simulink library "haley_test_bench_lib"  (Simulink 9.2)
settings: Solver=VariableStepAuto  StartTime=0.0  StopTime=10.0  RelTol=1e-3
undefined symbols (not defined in the file or in its folder): p_max_bar, t_sample_s
libraries: etherlab_lib x4, powerlib_meascontrol x2, simulink x1, pePwmGenerator x1
settings Model: Creator=habich  LastModifiedBy=entwicklungs-pc

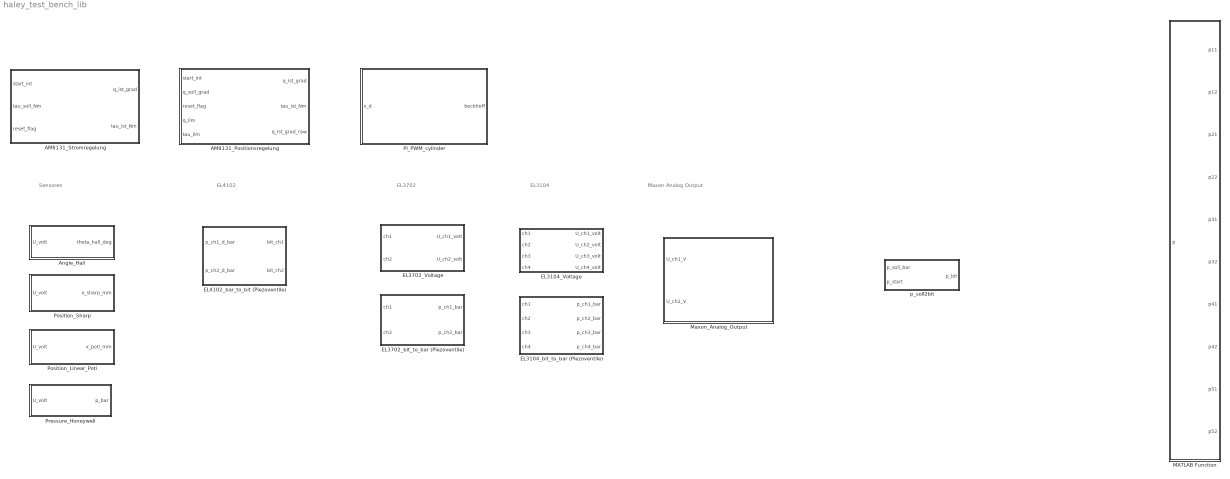
== system haley_test_bench_lib ==
  note: Sensoren
  note: EL4102
  note: EL3702
  note: Maxon Analog Output
  note: EL3104
  AM8131_Positionsregelung : Subsystem
  AM8131_Stromregelung : Subsystem
  Angle_Hall : MATLAB Function  TreatAsAtomicUnit=on
  EL3104_Voltage : Subsystem
  EL3104_bit_to_bar (Piezoventile) : Subsystem
  EL3702_Voltage : Subsystem
  EL3702_bit_to_bar (Piezoventile) : Subsystem
  EL4102_bar_to_bit (Piezoventile) : MATLAB Function  TreatAsAtomicUnit=on
  MATLAB Function : MATLAB Function  TreatAsAtomicUnit=on
  Maxon_Analog_Output : Subsystem
  PI_PWM_cylinder : Subsystem
  "Position_Linear_Poti " : MATLAB Function  TreatAsAtomicUnit=on
  Position_Sharp : MATLAB Function  TreatAsAtomicUnit=on
  Pressure_Honeywell : MATLAB Function  TreatAsAtomicUnit=on
  p_soll2bit : Subsystem

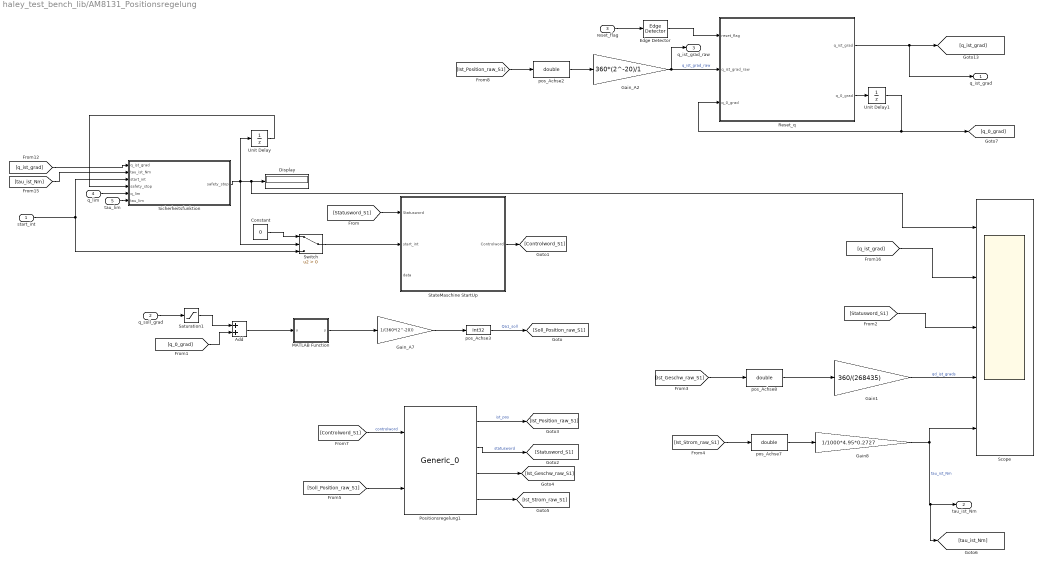
== system haley_test_bench_lib/AM8131_Positionsregelung ==
  start_int : Inport
  q_soll_grad : Inport  Port=2
  "reset_flag " : Inport  Port=3
  q_lim : Inport  Port=4
  tau_lim : Inport  Port=5
  Add : Sum
  Constant : Constant  Value=0
  Display : Display
  Edge Detector : powerlib_meascontrol/Logic/Edge Detector  model=Rising  ic=0  Ts=1e-3
      settings: SourceProductName=Simscape Electrical  SourceProductBaseCode=PS
  Gain1 : Gain  Gain=360/(268435)
  Gain8 : Gain  Gain=1/1000*4.95*0.2727
  Gain_A2 : Gain  Gain=360*(2^-20)/1
  Gain_A7 : Gain  Gain=1/(360*(2^-20))
  MATLAB Function : MATLAB Function  TreatAsAtomicUnit=on
  Positionsregelung1 : etherlab_lib/EtherCAT/Generic_0  master=0  index=6  rv=slave_el7211_pos  param=[]  tsample=0.001  debug=0
  Reset_q : MATLAB Function  TreatAsAtomicUnit=on
  Saturation1 : Saturate  UpperLimit=5  LowerLimit=-5
  Scope : Scope  NumInputPorts=5
  Sicherheitsfunktion : MATLAB Function  TreatAsAtomicUnit=on
  StateMaschine StartUp : Stateflow chart  TreatAsAtomicUnit=on
  Switch : Switch  Criteria=u2 > Threshold
  Unit Delay : UnitDelay  SampleTime=1e-3
  Unit Delay1 : UnitDelay  SampleTime=1e-3
  pos_Achse2 : DataTypeConversion  OutDataTypeStr=double
  pos_Achse3 : DataTypeConversion  OutDataTypeStr=int32
  pos_Achse7 : DataTypeConversion  OutDataTypeStr=double
  pos_Achse8 : DataTypeConversion  OutDataTypeStr=double
  "q_ist_grad " : Outport
  tau_ist_Nm : Outport  Port=2
  q_ist_grad_raw : Outport  Port=3
  wires:
  Positionsregelung1/1 -> [Ist_Position_raw_S1]  "ist_pos"
  [Statusword_S1] -> StateMaschine StartUp/1(Statusword)
  [Ist_Strom_raw_S1] -> pos_Achse7/1
  pos_Achse7/1 -> Gain8/1
  Positionsregelung1/2 -> [Statusword_S1]  "statusword"
  Gain8/1 -> [tau_ist_Nm], tau_ist_Nm/1, Scope/5  "tau_ist_Nm"
  StateMaschine StartUp/1(Controlword) -> [Controlword_S1]
  [Controlword_S1] -> Positionsregelung1/1  "controlword"
  [Statusword_S1] -> Scope/3
  Positionsregelung1/3 -> [Ist_Geschw_raw_S1]
  pos_Achse8/1 -> Gain1/1
  [Ist_Geschw_raw_S1] -> pos_Achse8/1
  Gain1/1 -> Scope/4  "qd_ist_grads"
  Positionsregelung1/4 -> [Ist_Strom_raw_S1]
  MATLAB Function/1(y) -> Gain_A7/1
  q_soll_grad/1 -> Saturation1/1
  Add/1 -> MATLAB Function/1(u)
  [Soll_Position_raw_S1] -> Positionsregelung1/2
  Gain_A7/1 -> pos_Achse3/1
  pos_Achse3/1 -> [Soll_Position_raw_S1]  "Qa1_soll"
  Reset_q/1(q_ist_grad) -> "q_ist_grad "/1, [q_ist_grad]
  [Ist_Position_raw_S1] -> pos_Achse2/1
  "reset_flag "/1 -> Edge Detector/1
  Edge Detector/1 -> Reset_q/1(reset_flag)
  Gain_A2/1 -> Reset_q/2(q_ist_grad_raw), q_ist_grad_raw/1  "q_ist_grad_raw"
  Reset_q/2(q_0_grad) -> Unit Delay1/1
  pos_Achse2/1 -> Gain_A2/1
  Unit Delay1/1 -> Reset_q/3("q_0_grad "), [q_0_grad]
  [q_ist_grad] -> Scope/2
  Unit Delay/1 -> Sicherheitsfunktion/4("safety_stop ")
  [q_ist_grad] -> Sicherheitsfunktion/1(q_ist_grad)
  Constant/1 -> Switch/1
  start_int/1 -> Switch/3, Sicherheitsfunktion/3(start_int)
  Sicherheitsfunktion/1(safety_stop) -> Scope/1, Display/1, Switch/2, Unit Delay/1
  [tau_ist_Nm] -> Sicherheitsfunktion/2(tau_ist_Nm)
  Switch/1 -> StateMaschine StartUp/2(start_int)
  [q_0_grad] -> Add/2
  Saturation1/1 -> Add/1
  q_lim/1 -> Sicherheitsfunktion/5(q_lim)
  tau_lim/1 -> Sicherheitsfunktion/6(tau_lim)

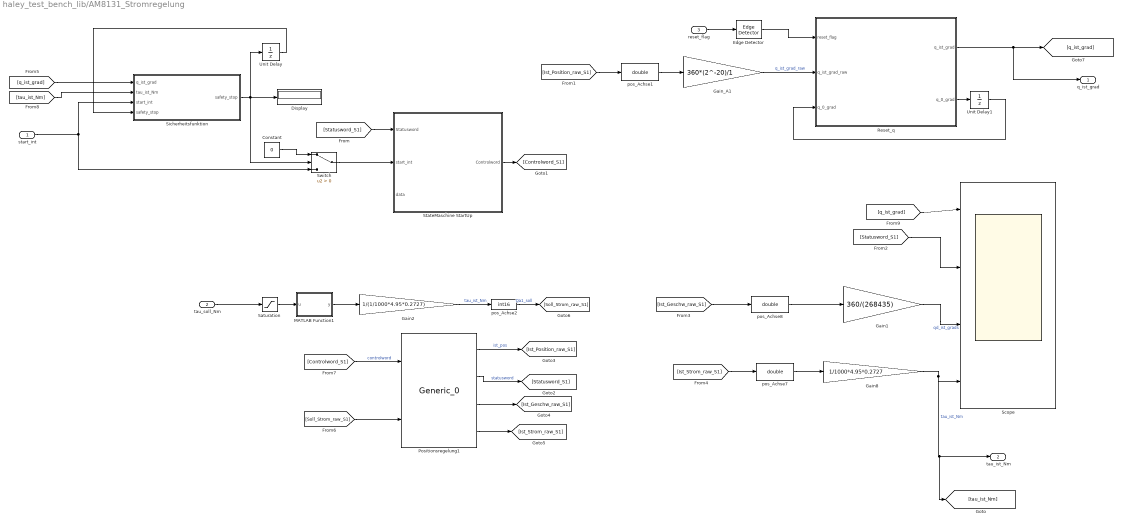
== system haley_test_bench_lib/AM8131_Stromregelung ==
  start_int : Inport
  tau_soll_Nm : Inport  Port=2
  "reset_flag " : Inport  Port=3
  Constant : Constant  Value=0
  Display : Display
  Edge Detector : powerlib_meascontrol/Logic/Edge Detector  model=Rising  ic=0  Ts=1e-3
      settings: SourceProductName=Simscape Electrical  SourceProductBaseCode=PS
  Gain1 : Gain  Gain=360/(268435)
  Gain2 : Gain  Gain=1/(1/1000*4.95*0.2727)
  Gain8 : Gain  Gain=1/1000*4.95*0.2727
  Gain_A1 : Gain  Gain=360*(2^-20)/1
  MATLAB Function1 : MATLAB Function  TreatAsAtomicUnit=on
  Positionsregelung1 : etherlab_lib/EtherCAT/Generic_0  master=0  index=6  rv=slave_el7211_strom  param=[]  tsample=0.001  debug=0
  Reset_q : MATLAB Function  TreatAsAtomicUnit=on
  Saturation : Saturate
  Scope : Scope  NumInputPorts=4
  Sicherheitsfunktion : MATLAB Function  TreatAsAtomicUnit=on
  StateMaschine StartUp : Stateflow chart  TreatAsAtomicUnit=on
  Switch : Switch  Criteria=u2 > Threshold
  Unit Delay : UnitDelay  SampleTime=1e-3
  Unit Delay1 : UnitDelay  SampleTime=1e-3
  pos_Achse1 : DataTypeConversion  OutDataTypeStr=double
  pos_Achse2 : DataTypeConversion  OutDataTypeStr=int16
  pos_Achse7 : DataTypeConversion  OutDataTypeStr=double
  pos_Achse8 : DataTypeConversion  OutDataTypeStr=double
  "q_ist_grad " : Outport
  "tau_ist_Nm " : Outport  Port=2
  wires:
  [Ist_Position_raw_S1] -> pos_Achse1/1
  Positionsregelung1/1 -> [Ist_Position_raw_S1]  "ist_pos"
  [Statusword_S1] -> StateMaschine StartUp/1(Statusword)
  [Ist_Strom_raw_S1] -> pos_Achse7/1
  pos_Achse7/1 -> Gain8/1
  MATLAB Function1/1(y) -> Gain2/1
  pos_Achse1/1 -> Gain_A1/1
  Positionsregelung1/2 -> [Statusword_S1]  "statusword"
  Gain8/1 -> [tau_ist_Nm], "tau_ist_Nm "/1, Scope/4  "tau_ist_Nm"
  StateMaschine StartUp/1(Controlword) -> [Controlword_S1]
  Saturation/1 -> MATLAB Function1/1(u)
  start_int/1 -> Switch/3, Sicherheitsfunktion/3(start_int)
  tau_soll_Nm/1 -> Saturation/1
  Gain2/1 -> pos_Achse2/1  "tau_ist_Nm"
  [Soll_Strom_raw_S1] -> Positionsregelung1/2
  [Controlword_S1] -> Positionsregelung1/1  "controlword"
  [Statusword_S1] -> Scope/2
  Positionsregelung1/3 -> [Ist_Geschw_raw_S1]
  pos_Achse8/1 -> Gain1/1
  [Ist_Geschw_raw_S1] -> pos_Achse8/1
  Gain1/1 -> Scope/3  "qd_ist_grads"
  Positionsregelung1/4 -> [Ist_Strom_raw_S1]
  pos_Achse2/1 -> [Soll_Strom_raw_S1]  "Qa1_soll"
  [q_ist_grad] -> Sicherheitsfunktion/1(q_ist_grad)
  [tau_ist_Nm] -> Sicherheitsfunktion/2(tau_ist_Nm)
  Sicherheitsfunktion/1(safety_stop) -> Display/1, Switch/2, Unit Delay/1
  Unit Delay/1 -> Sicherheitsfunktion/4("safety_stop ")
  Constant/1 -> Switch/1
  Switch/1 -> StateMaschine StartUp/2(start_int)
  Edge Detector/1 -> Reset_q/1(reset_flag)
  Gain_A1/1 -> Reset_q/2(q_ist_grad_raw)  "q_ist_grad_raw"
  Reset_q/2(q_0_grad) -> Unit Delay1/1
  Unit Delay1/1 -> Reset_q/3("q_0_grad ")
  Reset_q/1(q_ist_grad) -> "q_ist_grad "/1, [q_ist_grad]
  [q_ist_grad] -> Scope/1
  "reset_flag "/1 -> Edge Detector/1

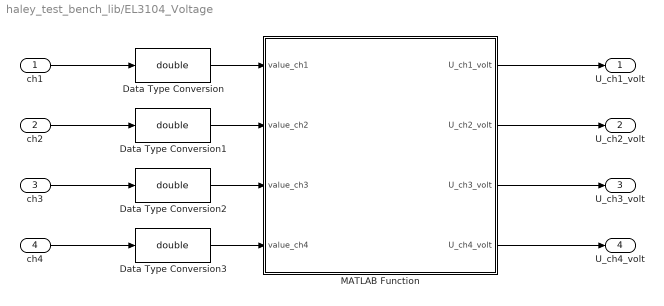
== system haley_test_bench_lib/EL3104_Voltage ==
  ch1 : Inport
  ch2 : Inport  Port=2
  ch3 : Inport  Port=3
  ch4 : Inport  Port=4
  Data Type Conversion{,1..3} (4 alike) : DataTypeConversion  OutDataTypeStr=double
  MATLAB Function : MATLAB Function  TreatAsAtomicUnit=on
  U_ch1_volt : Outport
  U_ch2_volt : Outport  Port=2
  U_ch3_volt : Outport  Port=3
  U_ch4_volt : Outport  Port=4
  wires:
  ch1/1 -> Data Type Conversion/1
  ch2/1 -> Data Type Conversion1/1
  Data Type Conversion1/1 -> MATLAB Function/2(value_ch2)
  MATLAB Function/2(U_ch2_volt) -> U_ch2_volt/1
  Data Type Conversion/1 -> MATLAB Function/1(value_ch1)
  MATLAB Function/1(U_ch1_volt) -> U_ch1_volt/1
  Data Type Conversion2/1 -> MATLAB Function/3(value_ch3)
  ch3/1 -> Data Type Conversion2/1
  Data Type Conversion3/1 -> MATLAB Function/4(value_ch4)
  ch4/1 -> Data Type Conversion3/1
  MATLAB Function/3(U_ch3_volt) -> U_ch3_volt/1
  MATLAB Function/4(U_ch4_volt) -> U_ch4_volt/1

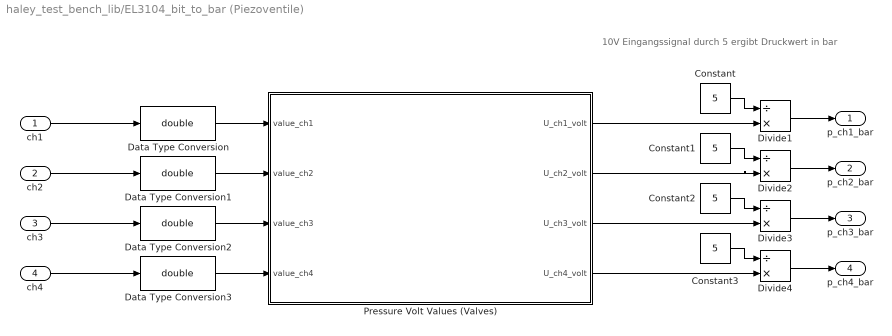
== system haley_test_bench_lib/EL3104_bit_to_bar (Piezoventile) ==
  note: 10V Eingangssignal durch 5 ergibt Druckwert in bar
  ch1 : Inport
  ch2 : Inport  Port=2
  ch3 : Inport  Port=3
  ch4 : Inport  Port=4
  Constant{,1..3} (4 alike) : Constant  Value=5
  Data Type Conversion{,1..3} (4 alike) : DataTypeConversion  OutDataTypeStr=double
  Divide{1..4} (4 alike) : Product  Inputs=/*
  Pressure Volt Values (Valves) : MATLAB Function  TreatAsAtomicUnit=on
  p_ch1_bar : Outport
  p_ch2_bar : Outport  Port=2
  p_ch3_bar : Outport  Port=3
  p_ch4_bar : Outport  Port=4
  wires:
  Pressure Volt Values (Valves)/1(U_ch1_volt) -> Divide1/2
  Constant/1 -> Divide1/1
  Data Type Conversion1/1 -> Pressure Volt Values (Valves)/2(value_ch2)
  Divide1/1 -> p_ch1_bar/1
  ch2/1 -> Data Type Conversion1/1
  ch1/1 -> Data Type Conversion/1
  Data Type Conversion/1 -> Pressure Volt Values (Valves)/1(value_ch1)
  Data Type Conversion2/1 -> Pressure Volt Values (Valves)/3(value_ch3)
  ch3/1 -> Data Type Conversion2/1
  Data Type Conversion3/1 -> Pressure Volt Values (Valves)/4(value_ch4)
  ch4/1 -> Data Type Conversion3/1
  Pressure Volt Values (Valves)/2(U_ch2_volt) -> Divide2/2
  Divide2/1 -> p_ch2_bar/1
  Constant1/1 -> Divide2/1
  Pressure Volt Values (Valves)/3(U_ch3_volt) -> Divide3/2
  Divide3/1 -> p_ch3_bar/1
  Constant2/1 -> Divide3/1
  Pressure Volt Values (Valves)/4(U_ch4_volt) -> Divide4/2
  Divide4/1 -> p_ch4_bar/1
  Constant3/1 -> Divide4/1

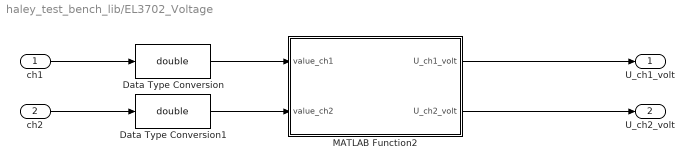
== system haley_test_bench_lib/EL3702_Voltage ==
  "ch1 " : Inport
  ch2 : Inport  Port=2
  Data Type Conversion : DataTypeConversion  OutDataTypeStr=double
  Data Type Conversion1 : DataTypeConversion  OutDataTypeStr=double
  MATLAB Function2 : MATLAB Function  TreatAsAtomicUnit=on
  U_ch1_volt : Outport
  U_ch2_volt : Outport  Port=2
  wires:
  MATLAB Function2/1(U_ch1_volt) -> U_ch1_volt/1
  Data Type Conversion1/1 -> MATLAB Function2/2(value_ch2)
  ch2/1 -> Data Type Conversion1/1
  "ch1 "/1 -> Data Type Conversion/1
  Data Type Conversion/1 -> MATLAB Function2/1(value_ch1)
  MATLAB Function2/2(U_ch2_volt) -> U_ch2_volt/1

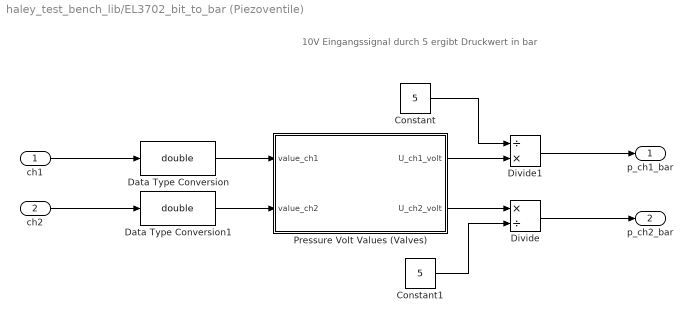
== system haley_test_bench_lib/EL3702_bit_to_bar (Piezoventile) ==
  note: 10V Eingangssignal durch 5 ergibt Druckwert in bar
  "ch1 " : Inport
  ch2 : Inport  Port=2
  Constant : Constant  Value=5
  Constant1 : Constant  Value=5
  Data Type Conversion : DataTypeConversion  OutDataTypeStr=double
  Data Type Conversion1 : DataTypeConversion  OutDataTypeStr=double
  Divide : Product  Inputs=*/
  Divide1 : Product  Inputs=/*
  Pressure Volt Values (Valves) : MATLAB Function  TreatAsAtomicUnit=on
  p_ch1_bar : Outport
  p_ch2_bar : Outport  Port=2
  wires:
  "ch1 "/1 -> Data Type Conversion/1
  Pressure Volt Values (Valves)/2(U_ch2_volt) -> Divide/1
  ch2/1 -> Data Type Conversion1/1
  Pressure Volt Values (Valves)/1(U_ch1_volt) -> Divide1/2
  Constant/1 -> Divide1/1
  Divide1/1 -> p_ch1_bar/1
  Divide/1 -> p_ch2_bar/1
  Constant1/1 -> Divide/2
  Data Type Conversion/1 -> Pressure Volt Values (Valves)/1(value_ch1)
  Data Type Conversion1/1 -> Pressure Volt Values (Valves)/2(value_ch2)

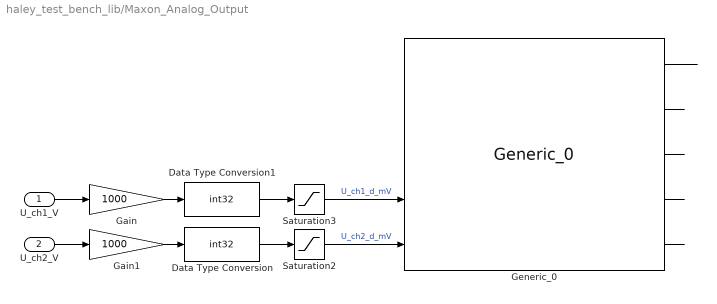
== system haley_test_bench_lib/Maxon_Analog_Output ==
  U_ch1_V : Inport
  U_ch2_V : Inport  Port=2
  Data Type Conversion : DataTypeConversion  OutDataTypeStr=int32
  Data Type Conversion1 : DataTypeConversion  OutDataTypeStr=int32
  Gain : Gain  Gain=1000
  Gain1 : Gain  Gain=1000
  Generic_0 : etherlab_lib/EtherCAT/Generic_0  master=0  index=9  rv=slave_io_maxon  param=[]  tsample=1e-3  debug=0
  Saturation2 : Saturate  UpperLimit=4000  LowerLimit=-4000
  Saturation3 : Saturate  UpperLimit=4000  LowerLimit=-4000
  wires:
  ? -> Generic_0/3
  Generic_0/1 -> ?
  Generic_0/3 -> ?
  ? -> Generic_0/2
  Gain1/1 -> Data Type Conversion/1
  Data Type Conversion/1 -> Saturation2/1
  Generic_0/4 -> ?
  Generic_0/5 -> ?
  ? -> Generic_0/1
  Saturation3/1 -> Generic_0/4  "U_ch1_d_mV"
  U_ch1_V/1 -> Gain/1
  Data Type Conversion1/1 -> Saturation3/1
  Generic_0/2 -> ?
  U_ch2_V/1 -> Gain1/1
  Gain/1 -> Data Type Conversion1/1
  Saturation2/1 -> Generic_0/5  "U_ch2_d_mV"

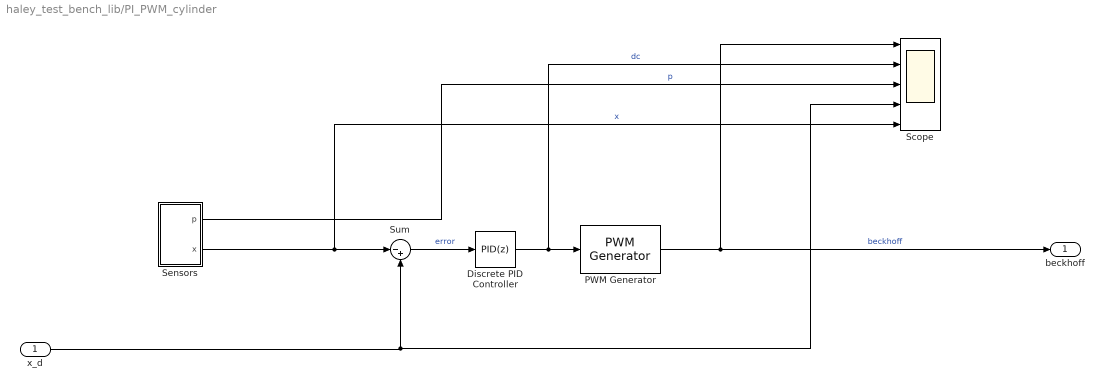
== system haley_test_bench_lib/PI_PWM_cylinder ==
  x_d : Inport
  Discrete PID Controller : simulink/Continuous/PID Controller  Controller=PID  Form=Ideal  TimeDomain=Discrete-time  SampleTime=1e-3  IntegratorMethod=Forward Euler  FilterMethod=Forward Euler  ControllerParametersSource=internal  P=0.07  I=2  D=0  UseFilter=on  N=100  TunerSelectOption=Transfer Function Based (PID Tuner App)  InitialConditionSource=internal  InitialConditionForIntegrator=0  InitialConditionForFilter=0  DifferentiatorICPrevScaledInput=0  ExternalReset=none  TrackingMode=off  Kt=1  LimitOutput=on  UpperSaturationLimit=0.9  LowerSaturationLimit=0.1  LinearizeAsGain=off  AntiWindupMode=clamping  Kb=100  POutMin=[]  POutMax=[]  IOutMin=[]  IOutMax=[]  DOutMin=[]  DOutMax=[]  NOutMin=[]  NOutMax=[]  SumOutMin=[]  SumOutMax=[]  SaturationOutMin=[]  SaturationOutMax=[]  PParamMin=[]  PParamMax=[]  IParamMin=[]  IParamMax=[]  DParamMin=[]  DParamMax=[]  NParamMin=[]  NParamMax=[]  KbParamMin=[]  KbParamMax=[]  KtParamMin=[]  KtParamMax=[]  KbOutMin=[]  KbOutMax=[]  KtOutMin=[]  KtOutMax=[]  IntegratorOutMin=[]  IntegratorOutMax=[]  FilterOutMin=[]  FilterOutMax=[]  SumI1OutMin=[]  SumI1OutMax=[]  SumI2OutMin=[]  SumI2OutMax=[]  SumI3OutMin=[]  SumI3OutMax=[]  SumI4OutMin=[]  SumI4OutMax=[]  SumDOutMin=[]  SumDOutMax=[]  DifferentiatorOutMin=[]  DifferentiatorOutMax=[]  FilterDiffOutCoefMin=[]  FilterDiffOutCoefMax=[]  ReciprocalOutMin=[]  ReciprocalOutMax=[]  SumDenOutMin=[]  SumDenOutMax=[]  SumNumOutMin=[]  SumNumOutMax=[]  DivideOutMin=[]  DivideOutMax=[]  IntegratorContinuousStateAttributes=''  IntegratorStateMustResolveToSignalObject=off  IntegratorRTWStateStorageClass=Auto  FilterContinuousStateAttributes=''  FilterStateMustResolveToSignalObject=off  FilterRTWStateStorageClass=Auto  ParallelPVariant=Passthrough  IdealPVariant=InternalParameters  IVariant=InternalParameters  DVariant=InternalParameters  IntegratorVariant=Discrete  SatVariant=Enabled  AWVariant=DiscClampingIdeal  PCopyVariant=InternalParamsIdeal  TRVariant=Disabled  FdbkBlocksVariant=Forward  IdealPFdbkVariant=Disabled  SatFdbkVariant=Disabled  DerivativeFilterVariant=ForwardEulerFilter  NVariant=InternalParameters  NCopyVariant=Disabled  FilterICVariant=InternalICsFilter  IntegratorICVariant=InternalICs  ExternalResetVariant=Disabled  TRSumVariant=Passthrough  SumFdbkVariant=Disabled  SumVariant=Sum_PID
  PWM Generator : pePwmGenerator/PWM Generator  CarrCount=Up  Tper=20e-3  Ts=1e-4
  Scope : Scope  NumInputPorts=5
  Sensors : Subsystem
  Sum : Sum  Inputs=|-+
  beckhoff : Outport
  wires:
  Sum/1 -> Discrete PID Controller/1  "error"
  Sensors/1(p) -> Scope/3  "p"
  x_d/1 -> Scope/4, Sum/2
  PWM Generator/1 -> beckhoff/1, Scope/1  "beckhoff"
  Discrete PID Controller/1 -> Scope/2, PWM Generator/1  "dc"
  Sensors/2(x) -> Scope/5, Sum/1  "x"

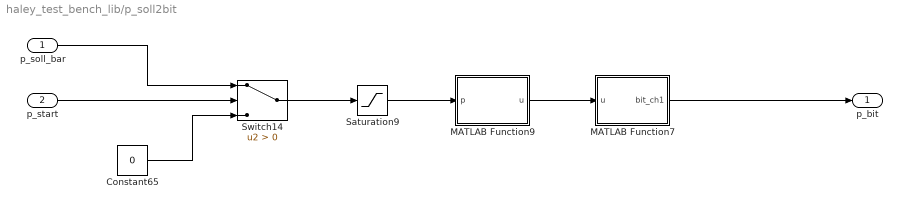
== system haley_test_bench_lib/p_soll2bit ==
  p_soll_bar : Inport
  p_start : Inport  Port=2
  Constant65 : Constant  Value=0  SampleTime=t_sample_s
  MATLAB Function7 : MATLAB Function  TreatAsAtomicUnit=on
  MATLAB Function9 : MATLAB Function  TreatAsAtomicUnit=on
  Saturation9 : Saturate  UpperLimit=p_max_bar  LowerLimit=0
  Switch14 : Switch  Criteria=u2 > Threshold
  p_bit : Outport
  wires:
  Switch14/1 -> Saturation9/1
  Constant65/1 -> Switch14/3
  Saturation9/1 -> MATLAB Function9/1(p)
  p_soll_bar/1 -> Switch14/1
  MATLAB Function7/1(bit_ch1) -> p_bit/1
  MATLAB Function9/1(u) -> MATLAB Function7/1(u)
  p_start/1 -> Switch14/2

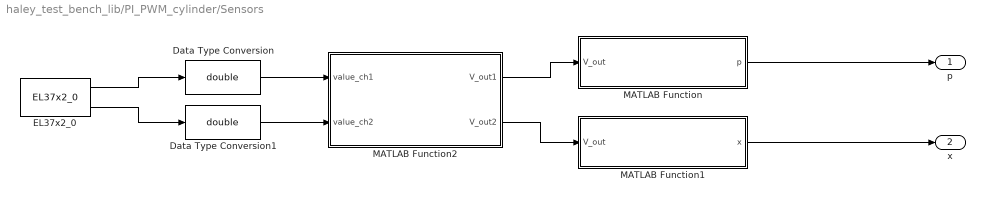
== system haley_test_bench_lib/PI_PWM_cylinder/Sensors ==
  Data Type Conversion : DataTypeConversion  OutDataTypeStr=double
  Data Type Conversion1 : DataTypeConversion  OutDataTypeStr=double
  EL37x2_0 : etherlab_lib/EtherCAT/Beckhoff/EL37x2_0  master=0  index=1  model=EL3702  revision=[242626642 131072]  one_ch=off  scale=[]  offset=[]  tsample=1e-3  debug=0  dc_mode=1  dc_assign_activate=hex2dec('730')  dc_cycle0=0  dc_cycle0_factor="-10     % 10-times OS"  dc_shift0=-10000  dc_shift0_factor=1  dc_shift0_input=off  dc_cycle1=0  dc_cycle1_factor=-1  dc_shift1=0  dc_shift1_factor=0
  MATLAB Function : MATLAB Function  TreatAsAtomicUnit=on
  MATLAB Function1 : MATLAB Function  TreatAsAtomicUnit=on
  MATLAB Function2 : MATLAB Function  TreatAsAtomicUnit=on
  p : Outport
  x : Outport  Port=2
  wires:
  MATLAB Function/1(p) -> p/1
  MATLAB Function1/1(x) -> x/1
  Data Type Conversion1/1 -> MATLAB Function2/2(value_ch2)
  Data Type Conversion/1 -> MATLAB Function2/1(value_ch1)
  EL37x2_0/1 -> Data Type Conversion/1
  MATLAB Function2/1(V_out1) -> MATLAB Function/1(V_out)
  EL37x2_0/2 -> Data Type Conversion1/1
  MATLAB Function2/2(V_out2) -> MATLAB Function1/1(V_out)

== matlab function AM8131_Stromregelung/MATLAB Function1 ==
  data: u input double; y output double
function y = check_nan(u)
if isnan(sum(u))
    y=0;
else
    y=u;
end

== matlab function AM8131_Positionsregelung/MATLAB Function ==
  data: u input double; y output double
function y = check_nan(u)
if isnan(sum(u))
    y=0;
else
    y=u;
end

== matlab function PI_PWM_cylinder/Sensors/MATLAB Function ==
  data: V_out input double; p output double
function p = CalcPressure(V_out)
%SSCDANN100PAAA5 pressure sensor
V_supply=5.068;%volt
p_max=100;%psi
p_min=0;%psi
psitobar=0.06894757293178;%psi=#psitobar*bar

p_max=p_max*psitobar;
p_min=p_min*psitobar;
p=(V_out-0.1*V_supply)/(0.8*V_supply)*(p_max-p_min)+p_min;

== stateflow chart AM8131_Positionsregelung/StateMaschine StartUp ==
  note: State0: start is not set
      | SW=0:
      | CW=0
      |
      | State1: start is set
      | SW=0
      | CW=0
      |
      | State2: Initialize Drive
      | SW=104=1101000 : Quickstop(Inverse); Fault; Switch on disabled
      | CW: 128=1000000: Fault reset;
      |
      | State3: Enable Voltage
      | SW=96=1100000: Quickstop(Inverse); Switch on disabled
      | CW=6= 00000110:Enable Voltage; Quickstop(Inverse)
      |
      | State4: Enable Drive
      | SW=33=1000001: Quickstop(Inverse); Ready to switch on
      | CW=7=00000111: Enable Voltage; Quickstop(Inverse); Switch On
      |
      | State5:  Enabled
      | SW=35=1000011: Quickstop(Inverse); Ready to switch on ; Switched on
      | CW=15=00001111:Enable Voltage; Quickstop(Inverse); Switch On;Enable Operation
  state State0
    during:
    Controlword = 0;
  state State1
    during: Controlword = 0;
  state State2
    during: Controlword = 128;
  state State3
    during: Controlword = 6;
  note: 1 blinkt
      | 8,9,16 leuchtet
  state State4
    during: Controlword = 7;
  state State5
    during: Controlword = 15;
  (default) -> State0
  State4 -> State0 [order 2] : [start_int == 0]
  State3 -> State0 [order 2] : [start_int == 0]
  State5 -> State0 : [start_int == 0]
  State2 -> State0 [order 2] : [start_int == 0]
  State1 -> State0 [order 3] : [start_int == 0]
  State0 -> State1 : [ start_int == 1 ]
  State1 -> State3 [order 2] : [ Statusword == 96 ]
  State1 -> State2 [order 1] : [ Statusword == 104 ]
  State2 -> State3 [order 1] : [ Statusword == 96 ]
  State3 -> State4 [order 1] : [ Statusword == 33 ]
  State4 -> State5 [order 1] : [ Statusword == 35 ]
  data: Statusword input double; Controlword output double; start_int input double; data input double

== matlab function PI_PWM_cylinder/Sensors/MATLAB Function1 ==
  data: V_out input double; x output double
function x = CalcPosition(V_out)
%Linear Poti
V_min=0.038;%Volt Kolben eingefahren
V_max=2.671;%volt Kolben ausgefahren
x_max=50;%mm
x_min=0;%mm

%Linear
x=(V_out-V_min)*(x_max-x_min)/(V_max-V_min);%mm

== matlab function PI_PWM_cylinder/Sensors/MATLAB Function2 ==
  data: value_ch1 input double; V_out1 output double; value_ch2 input double; V_out2 output double
function [V_out1,V_out2] = BeckhoffToVoltage(value_ch1,value_ch2)
%Beckhoff EL3702 +-10V Analog Input 16 Bit
V_out1=10/32767*value_ch1;
V_out2=10/32767*value_ch2;

== matlab function Position_Linear_Poti  ==
  data: U_volt input double; x_poti_mm output double
function x_poti_mm = fcn(U_volt)
%Linear Poti
V_min=0.038;%Volt Kolben eingefahren
V_max=2.671;%volt Kolben ausgefahren
x_max=50;%mm
x_min=0;%mm

%Linear
x_poti_mm=(U_volt-V_min)*(x_max-x_min)/(V_max-V_min);%mm

== matlab function Pressure_Honeywell ==
  data: U_volt input double; p_bar output double
function p_bar = fcn(U_volt)
%SSCDANN100PAAA5 pressure sensor
V_supply=5.068;%volt
p_max=100;%psi
p_min=0;%psi
psitobar=0.06894757293178;%psi=#psitobar*bar

p_max=p_max*psitobar;
p_min=p_min*psitobar;
p_bar=(U_volt-0.1*V_supply)/(0.8*V_supply)*(p_max-p_min)+p_min;

== matlab function Position_Sharp ==
  data: U_volt input double; x_sharp_mm output double
function x_sharp_mm = fcn(U_volt)

x_sharp_mm =(2.0845*U_volt^6)-(23.244*U_volt^5)+(104.5*U_volt^4)-(244.01*U_volt^3)+(318.01*U_volt^2)-(231.32*U_volt)+87.061

== matlab function Angle_Hall ==
  data: U_volt input double; theta_hall_deg output double
function theta_hall_deg = fcn(U_volt)
theta_hall_deg= (U_volt*(1/9.99))*360

== matlab function EL3702_Voltage/MATLAB Function2 ==
  data: U_ch1_volt output double; value_ch1 input double; U_ch2_volt output double; value_ch2 input double
function [U_ch1_volt,U_ch2_volt] = BeckhoffToVoltage(value_ch1,value_ch2)
%Beckhoff EL3702 +-10V Analog Input 16 Bit
U_ch1_volt=10/32767*value_ch1;
U_ch2_volt=10/32767*value_ch2;

== matlab function AM8131_Stromregelung/Sicherheitsfunktion ==
  data: q_ist_grad input double; safety_stop output double; tau_ist_Nm input double; start_int input double; safety_stop input double
function safety_stop = fcn(q_ist_grad,tau_ist_Nm,start_int,safety_stop)
if safety_stop
    % hold
    safety_stop=1;
elseif start_int==1 && ((q_ist_grad>5 || q_ist_grad<-5) || (tau_ist_Nm>0.5 || tau_ist_Nm<-0.5))
    safety_stop=1;
else
    safety_stop=0;
end

== matlab function AM8131_Stromregelung/Reset_q ==
  data: reset_flag input double; q_ist_grad_raw input double; q_ist_grad output double; q_0_grad input double; q_0_grad output double
function [q_ist_grad,q_0_grad] = fcn(reset_flag,q_ist_grad_raw,q_0_grad)
if reset_flag
    q_0_grad=q_ist_grad_raw;
end
q_ist_grad=q_ist_grad_raw-q_0_grad;

== matlab function EL4102_bar_to_bit (Piezoventile) ==
  data: p_ch1_d_bar input double; bit_ch1 output double; p_ch2_d_bar input double; bit_ch2 output double
function [bit_ch1,bit_ch2]= bar_to_bit(p_ch1_d_bar,p_ch2_d_bar)

Volt_1 = p_ch1_d_bar*5; %Umrechnung des Druckwerts(bar) in Volt
Volt_2 = p_ch2_d_bar*5;

bit_ch1=Volt_1/10*32767; %10V in Bit umrechnen
bit_ch2=Volt_2/10*32767;

== matlab function AM8131_Positionsregelung/Reset_q ==
  data: reset_flag input double; q_ist_grad_raw input double; q_ist_grad output double; q_0_grad input double; q_0_grad output double
function [q_ist_grad,q_0_grad] = fcn(reset_flag,q_ist_grad_raw,q_0_grad)
if reset_flag
    q_0_grad=q_ist_grad_raw;
end
q_ist_grad=q_ist_grad_raw-q_0_grad;

== matlab function AM8131_Positionsregelung/Sicherheitsfunktion ==
  data: q_ist_grad input double; safety_stop output double; tau_ist_Nm input double; start_int input double; safety_stop input double; q_lim input double; tau_lim input double
function safety_stop = fcn(q_ist_grad,tau_ist_Nm,start_int,safety_stop, q_lim, tau_lim)
if safety_stop
    % hold
    safety_stop=1;
elseif start_int==1 && ((q_ist_grad>abs(q_lim) || q_ist_grad<-1*abs(q_lim)) || (tau_ist_Nm>abs(tau_lim) || tau_ist_Nm<-1*abs(tau_lim)))
    safety_stop=1;
else
    safety_stop=0;
end

== matlab function EL3104_bit_to_bar (Piezoventile)/Pressure Volt Values (Valves) ==
  data: value_ch1 input double; U_ch1_volt output double; value_ch2 input double; value_ch3 input double; value_ch4 input double; U_ch2_volt output double; U_ch3_volt output double; U_ch4_volt output double
function [U_ch1_volt,U_ch2_volt,U_ch3_volt,U_ch4_volt] = BeckhoffToVoltage(value_ch1,value_ch2,value_ch3,value_ch4)
%Beckhoff EL3104 +-10V Analog Input 16 Bit
U_ch1_volt=10/32767*value_ch1;
U_ch2_volt=10/32767*value_ch2;
U_ch3_volt=10/32767*value_ch3;
U_ch4_volt=10/32767*value_ch4;

== matlab function EL3702_bit_to_bar (Piezoventile)/Pressure Volt Values (Valves) ==
  data: U_ch1_volt output double; value_ch1 input double; U_ch2_volt output double; value_ch2 input double
function [U_ch1_volt,U_ch2_volt] = BeckhoffToVoltage(value_ch1,value_ch2)
%Beckhoff EL3702 +-10V Analog Input 16 Bit
U_ch1_volt=10/32767*value_ch1;
U_ch2_volt=10/32767*value_ch2;

== matlab function EL3104_Voltage/MATLAB Function ==
  data: value_ch1 input double; U_ch1_volt output double; value_ch2 input double; U_ch2_volt output double; value_ch3 input double; value_ch4 input double; U_ch3_volt output double; U_ch4_volt output double
function [U_ch1_volt,U_ch2_volt,U_ch3_volt,U_ch4_volt] = BeckhoffToVoltage3104(value_ch1,value_ch2,value_ch3,value_ch4)
%Beckhoff EL3104 +-10V Analog Input 16 Bit
U_ch1_volt=10/32767*value_ch1;
U_ch2_volt=10/32767*value_ch2;
U_ch3_volt=10/32767*value_ch3;
U_ch4_volt=10/32767*value_ch4;

== matlab function MATLAB Function ==
  data: p input double; p11 output double; p12 output double; p21 output double; p22 output double; p31 output double; p32 output double; p41 output double; p42 output double; p51 output double; p52 output double
function [p11,p12,p21,p22,p31,p32,p41,p42,p51,p52]= pvec2scalar(p)
p11=p(1);
p12=p(2);
p21=p(3);
p22=p(4);
p31=p(5);
p32=p(6);
p41=p(7);
p42=p(8);
p51=p(9);
p52=p(10);

== matlab function p_soll2bit/MATLAB Function7 ==
  data: u input double; bit_ch1 output double
function bit_ch1 = fcn(u)
bit_ch1=u/10*32768; %10V in 16 Bit signed Int umrechnen, obwohl Klemme nur 12 Bit Aufl�sung hat (siehe Datenblatt)

== matlab function p_soll2bit/MATLAB Function9 ==
  data: p input double; u output double
function u = fcn(p)
    u = 0;
    if p<=2 %p_max = 2bar
        u= p*5; %Umrechnung des Druckwerts(bar) in Volt
    end
end

== stateflow chart AM8131_Stromregelung/StateMaschine StartUp ==
  note: State0: start is not set
      | SW=0:
      | CW=0
      |
      | State1: start is set
      | SW=0
      | CW=0
      |
      | State2: Initialize Drive
      | SW=104=1101000 : Quickstop(Inverse); Fault; Switch on disabled
      | CW: 128=1000000: Fault reset;
      |
      | State3: Enable Voltage
      | SW=96=1100000: Quickstop(Inverse); Switch on disabled
      | CW=6= 00000110:Enable Voltage; Quickstop(Inverse)
      |
      | State4: Enable Drive
      | SW=33=1000001: Quickstop(Inverse); Ready to switch on
      | CW=7=00000111: Enable Voltage; Quickstop(Inverse); Switch On
      |
      | State5:  Enabled
      | SW=35=1000011: Quickstop(Inverse); Ready to switch on ; Switched on
      | CW=15=00001111:Enable Voltage; Quickstop(Inverse); Switch On;Enable Operation
  state State0
    during:
    Controlword = 0;
  state State1
    during: Controlword = 0;
  state State2
    during: Controlword = 128;
  state State3
    during: Controlword = 6;
  note: 1 blinkt
      | 8,9,16 leuchtet
  state State4
    during: Controlword = 7;
  state State5
    during: Controlword = 15;
  (default) -> State0
  State4 -> State0 [order 2] : [start_int == 0]
  State3 -> State0 [order 2] : [start_int == 0]
  State5 -> State0 : [start_int == 0]
  State2 -> State0 [order 2] : [start_int == 0]
  State1 -> State0 [order 3] : [start_int == 0]
  State0 -> State1 : [ start_int == 1 ]
  State1 -> State3 [order 2] : [ Statusword == 96 ]
  State1 -> State2 [order 1] : [ Statusword == 104 ]
  State2 -> State3 [order 1] : [ Statusword == 96 ]
  State3 -> State4 [order 1] : [ Statusword == 33 ]
  State4 -> State5 [order 1] : [ Statusword == 35 ]
  data: Statusword input double; Controlword output double; start_int input double; data input double
